simulink model "DC_CL_simu_PlotRealtime"  (R2017a)
settings: Solver=ode45  StartTime=0.0  StopTime=inf  RelTol=1e-3  EnableMultiTasking=on
InitFcn:
  | init_DC_param;
undefined symbols (not defined in the file or in its folder): Busy, param, Wait
libraries: simulink x3, aerolibanimutils x2
settings Model: Creator=Messn  LastModifiedBy=messn
settings DataIOCC: SaveFormat=Array  SaveOutput=off  TimeSaveName=t  Refine=3
settings OptimizationCC: ExpressionDepthLimit=2147483647  LifeSpan=inf
settings DebuggingCC: UnderspecifiedInitializationDetection=Classic  MergeDetectMultiDrivingBlocksExec=none  StateNameClashWarn=warning  SFUnexpectedBacktrackingDiag=warning  SFNoUnconditionalDefaultTransitionDiag=warning  SFExecutionAtInitializationDiag=none
settings HardwareCC: ProdBitPerPointer=32  ProdBitPerSizeT=32  ProdBitPerPtrDiffT=32  ProdLargestAtomicFloat=None  ProdIntDivRoundTo=Undefined  ProdEndianess=Unspecified  ProdWordSize=32  ProdHWDeviceType=32-bit Generic
settings ModelReferenceCC: PropagateSignalLabelsOutOfModel=off
settings GRTTargetCC: TargetLangStandard=C89/C90 (ANSI)  GeneratePreprocessorConditionals=Disable all
settings ConfigComp: CovMetricSettings=dw  CovHtmlReporting=on  CovSaveCumulativeToWorkspaceVar=on  CovSaveSingleToWorkspaceVar=on  CovExternalEMLEnable=off  CovSFcnEnable=off

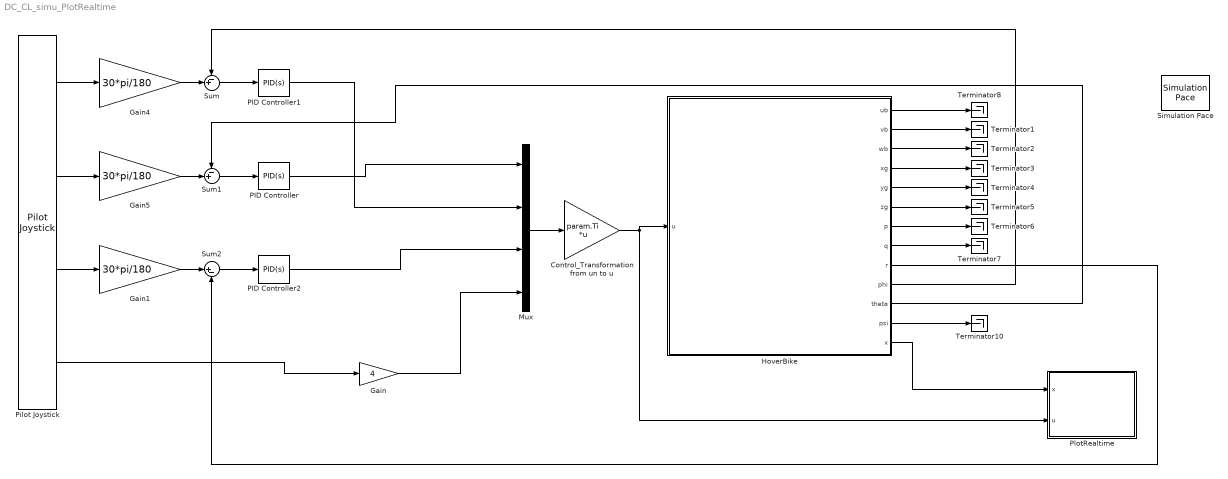
== system DC_CL_simu_PlotRealtime ==
  Control_Transformation from un to u : Gain  Gain=param.Ti  Multiplication=Matrix(K*u)
  Gain : Gain  Gain=4
  Gain1 : Gain  Gain=30*pi/180
  Gain4 : Gain  Gain=30*pi/180
  Gain5 : Gain  Gain=30*pi/180
  HoverBike : Subsystem
  Mux : Mux
  PID Controller : simulink/Continuous/PID Controller  Controller=PID  TimeDomain=Continuous-time  SampleTime=-1  IntegratorMethod=Forward Euler  FilterMethod=Forward Euler  Form=Parallel  UseFilter=on  ControllerParametersSource=internal  P=-0.119609159457863  I=-0.0298872891132111  D=-0.0962817830854201  N=11.7108788988861  InitialConditionSource=internal  InitialConditionForIntegrator=0  InitialConditionForFilter=0  ExternalReset=none  LimitOutput=off  UpperSaturationLimit=inf  LowerSaturationLimit=-inf  LinearizeAsGain=on  AntiWindupMode=none  Kb=1  TrackingMode=off  Kt=1  PParamMin=[]  PParamMax=[]  IParamMin=[]  IParamMax=[]  DParamMin=[]  DParamMax=[]  NParamMin=[]  NParamMax=[]  KbParamMin=[]  KbParamMax=[]  KtParamMin=[]  KtParamMax=[]  POutMin=[]  POutMax=[]  IOutMin=[]  IOutMax=[]  DOutMin=[]  DOutMax=[]  NOutMin=[]  NOutMax=[]  KbOutMin=[]  KbOutMax=[]  KtOutMin=[]  KtOutMax=[]  IntegratorOutMin=[]  IntegratorOutMax=[]  FilterOutMin=[]  FilterOutMax=[]  SumOutMin=[]  SumOutMax=[]  SumI1OutMin=[]  SumI1OutMax=[]  SumI2OutMin=[]  SumI2OutMax=[]  SumI3OutMin=[]  SumI3OutMax=[]  SumDOutMin=[]  SumDOutMax=[]  SaturationOutMin=[]  SaturationOutMax=[]  IntegratorContinuousStateAttributes=''  IntegratorStateMustResolveToSignalObject=off  IntegratorRTWStateStorageClass=Auto  FilterContinuousStateAttributes=''  FilterStateMustResolveToSignalObject=off  FilterRTWStateStorageClass=Auto  DifferentiatorICPrevScaledInput=0  DifferentiatorOutMin=[]  DifferentiatorOutMax=[]  InitialConditionSetting=State (most efficient)
  PID Controller1 : simulink/Continuous/PID Controller  Controller=PID  TimeDomain=Continuous-time  SampleTime=-1  IntegratorMethod=Forward Euler  FilterMethod=Forward Euler  Form=Parallel  UseFilter=on  ControllerParametersSource=internal  P=0.00835714838010559  I=0.00107403388129509  D=0.0149858292850059  N=9.73667034237561  InitialConditionSource=internal  InitialConditionForIntegrator=0  InitialConditionForFilter=0  ExternalReset=none  LimitOutput=off  UpperSaturationLimit=inf  LowerSaturationLimit=-inf  LinearizeAsGain=on  AntiWindupMode=none  Kb=1  TrackingMode=off  Kt=1  PParamMin=[]  PParamMax=[]  IParamMin=[]  IParamMax=[]  DParamMin=[]  DParamMax=[]  NParamMin=[]  NParamMax=[]  KbParamMin=[]  KbParamMax=[]  KtParamMin=[]  KtParamMax=[]  POutMin=[]  POutMax=[]  IOutMin=[]  IOutMax=[]  DOutMin=[]  DOutMax=[]  NOutMin=[]  NOutMax=[]  KbOutMin=[]  KbOutMax=[]  KtOutMin=[]  KtOutMax=[]  IntegratorOutMin=[]  IntegratorOutMax=[]  FilterOutMin=[]  FilterOutMax=[]  SumOutMin=[]  SumOutMax=[]  SumI1OutMin=[]  SumI1OutMax=[]  SumI2OutMin=[]  SumI2OutMax=[]  SumI3OutMin=[]  SumI3OutMax=[]  SumDOutMin=[]  SumDOutMax=[]  SaturationOutMin=[]  SaturationOutMax=[]  IntegratorContinuousStateAttributes=''  IntegratorStateMustResolveToSignalObject=off  IntegratorRTWStateStorageClass=Auto  FilterContinuousStateAttributes=''  FilterStateMustResolveToSignalObject=off  FilterRTWStateStorageClass=Auto  DifferentiatorICPrevScaledInput=0  DifferentiatorOutMin=[]  DifferentiatorOutMax=[]  InitialConditionSetting=State (most efficient)
  PID Controller2 : simulink/Continuous/PID Controller  Controller=PID  TimeDomain=Continuous-time  SampleTime=-1  IntegratorMethod=Forward Euler  FilterMethod=Forward Euler  Form=Parallel  UseFilter=on  ControllerParametersSource=internal  P=0.116001216751594  I=0.0498672968614691  D=-0.0125507347856546  N=2.65016683380004  InitialConditionSource=internal  InitialConditionForIntegrator=0  InitialConditionForFilter=0  ExternalReset=none  LimitOutput=off  UpperSaturationLimit=inf  LowerSaturationLimit=-inf  LinearizeAsGain=on  AntiWindupMode=none  Kb=1  TrackingMode=off  Kt=1  PParamMin=[]  PParamMax=[]  IParamMin=[]  IParamMax=[]  DParamMin=[]  DParamMax=[]  NParamMin=[]  NParamMax=[]  KbParamMin=[]  KbParamMax=[]  KtParamMin=[]  KtParamMax=[]  POutMin=[]  POutMax=[]  IOutMin=[]  IOutMax=[]  DOutMin=[]  DOutMax=[]  NOutMin=[]  NOutMax=[]  KbOutMin=[]  KbOutMax=[]  KtOutMin=[]  KtOutMax=[]  IntegratorOutMin=[]  IntegratorOutMax=[]  FilterOutMin=[]  FilterOutMax=[]  SumOutMin=[]  SumOutMax=[]  SumI1OutMin=[]  SumI1OutMax=[]  SumI2OutMin=[]  SumI2OutMax=[]  SumI3OutMin=[]  SumI3OutMax=[]  SumDOutMin=[]  SumDOutMax=[]  SaturationOutMin=[]  SaturationOutMax=[]  IntegratorContinuousStateAttributes=''  IntegratorStateMustResolveToSignalObject=off  IntegratorRTWStateStorageClass=Auto  FilterContinuousStateAttributes=''  FilterStateMustResolveToSignalObject=off  FilterRTWStateStorageClass=Auto  DifferentiatorICPrevScaledInput=0  DifferentiatorOutMin=[]  DifferentiatorOutMax=[]  InitialConditionSetting=State (most efficient)
  Pilot Joystick : aerolibanimutils/Pilot Joystick  JoystickID=Joystick1  OutputConfiguration=FourAxis  SampleTime=1/30
  PlotRealtime : Subsystem
  Simulation Pace : aerolibanimutils/Simulation Pace  SimulationPace=1  SleepMode=Busy-Wait  OutputPaceError=off  SampleTime=1/30
  Sum : Sum  Inputs=-+|
  Sum1 : Sum  Inputs=-+|
  Sum2 : Sum  Inputs=|+-
  Terminator{1..8,10} (9 alike) : Terminator
  wires:
  Control_Transformation from un to u/1 -> HoverBike/1(u), PlotRealtime/2(u)
  Pilot Joystick/1 -> Gain4/1
  Pilot Joystick/4 -> Gain/1
  Mux/1 -> Control_Transformation from un to u/1
  Gain/1 -> Mux/4
  PID Controller1/1 -> Mux/2
  HoverBike/13(x) -> PlotRealtime/1(x)
  HoverBike/2(vb) -> Terminator1/1
  HoverBike/3(wb) -> Terminator2/1
  HoverBike/4(xg) -> Terminator3/1
  HoverBike/5(yg) -> Terminator4/1
  HoverBike/6(zg) -> Terminator5/1
  HoverBike/7(p) -> Terminator6/1
  HoverBike/8(q) -> Terminator7/1
  HoverBike/10(phi) -> Sum/1
  Sum/1 -> PID Controller1/1
  Gain4/1 -> Sum/2
  HoverBike/12(psi) -> Terminator10/1
  PID Controller/1 -> Mux/1
  HoverBike/11(theta) -> Sum1/1
  Sum1/1 -> PID Controller/1
  Gain5/1 -> Sum1/2
  Sum2/1 -> PID Controller2/1
  PID Controller2/1 -> Mux/3
  Gain1/1 -> Sum2/1
  HoverBike/9(r) -> Sum2/2
  Pilot Joystick/2 -> Gain5/1
  Pilot Joystick/3 -> Gain1/1
  HoverBike/1(ub) -> Terminator8/1

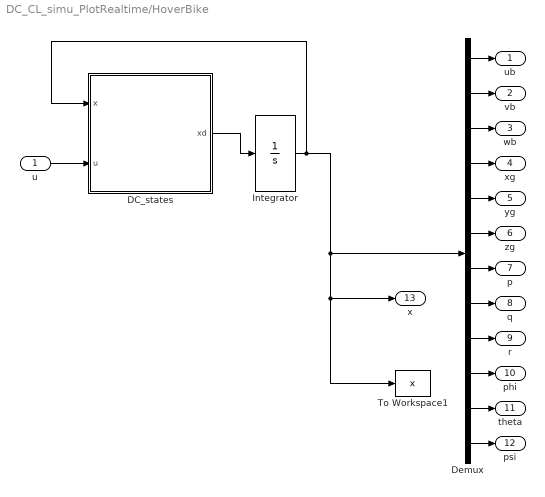
== system DC_CL_simu_PlotRealtime/HoverBike ==
  u : Inport
  DC_states : MATLAB Function  TreatAsAtomicUnit=on
  Demux : Demux  Outputs=12
  Integrator : Integrator
  To Workspace1 : ToWorkspace  VariableName=x  SampleTime=-1
  ub : Outport
  vb : Outport  Port=2
  wb : Outport  Port=3
  xg : Outport  Port=4
  yg : Outport  Port=5
  zg : Outport  Port=6
  p : Outport  Port=7
  q : Outport  Port=8
  r : Outport  Port=9
  phi : Outport  Port=10
  theta : Outport  Port=11
  psi : Outport  Port=12
  x : Outport  Port=13
  wires:
  u/1 -> DC_states/2(u)
  DC_states/1(xd) -> Integrator/1
  Integrator/1 -> DC_states/1(x), x/1, To Workspace1/1, Demux/1
  Demux/1 -> ub/1
  Demux/2 -> vb/1
  Demux/3 -> wb/1
  Demux/4 -> xg/1
  Demux/5 -> yg/1
  Demux/6 -> zg/1
  Demux/7 -> p/1
  Demux/8 -> q/1
  Demux/9 -> r/1
  Demux/10 -> phi/1
  Demux/11 -> theta/1
  Demux/12 -> psi/1

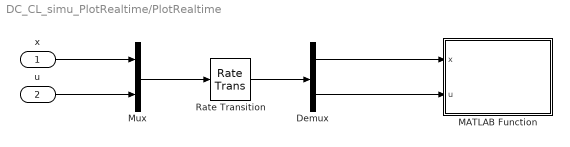
== system DC_CL_simu_PlotRealtime/PlotRealtime ==
  x : Inport
  u : Inport  Port=2
  Demux : Demux  Outputs=[12,4]
  MATLAB Function : MATLAB Function  InitFcn=init_PlotMultiCopter_Realtime  TreatAsAtomicUnit=on
  Mux : Mux  Inputs=2
  Rate Transition : RateTransition  OutPortSampleTime=0.1
  wires:
  Demux/2 -> MATLAB Function/2(u)
  x/1 -> Mux/1
  u/1 -> Mux/2
  Mux/1 -> Rate Transition/1
  Demux/1 -> MATLAB Function/1(x)
  Rate Transition/1 -> Demux/1

== matlab function DC_CL_simu_PlotRealtime/PlotRealtime/MATLAB Function ==
  data: x input; u input
function plotWrapper(x,u)

% This wrapper is used to exclude the 
% function "plot_MultiCopter_Realtime(x,u)" from
% the simulink compiler

coder.extrinsic('plot_MultiCopter_Realtime')
plot_MultiCopter_Realtime(x,u)

== matlab function DC_CL_simu_PlotRealtime/HoverBike/DC_states ==
  data: x input; u input; xd output size=12; param parameter
function xd = DC_states(x,u,param)
%#codegen
% Wrapper function that calculates state derivatives of a dualcopter 
% Author: Bernd Messnarz, Last Revision: 2017|04|06
xd = DC_dyn(0,x,u,param);
